simulink subsystem "NoVCU"  (R2024a)
settings: Solver=VariableStepAuto  StartTime=0.0  StopTime=10.0  RelTol=1e-3
settings Model: Creator=The MathWorks, Inc.  LastModifiedBy=The MathWorks, Inc.
settings RTWCC: GPUComputeCapability=3.5

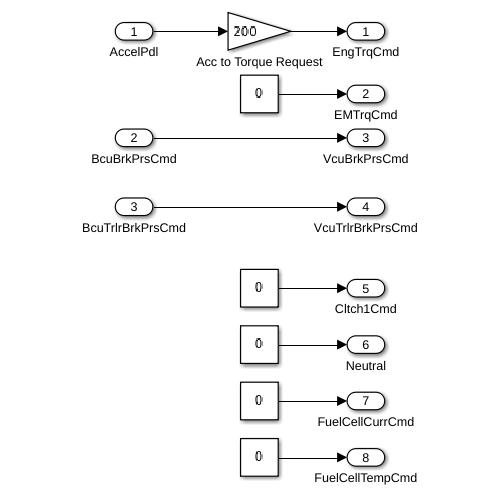
[thumbnail: Simulink's stored preview of the top-level diagram]
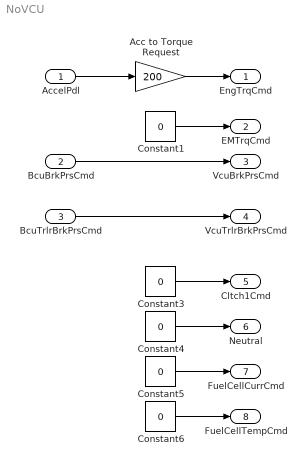
== system NoVCU ==
  AccelPdl : Inport
  BcuBrkPrsCmd : Inport  Port=2  SampleTime=0.01
  BcuTrlrBrkPrsCmd : Inport  Port=3  SampleTime=0.01
  Acc to Torque Request : Gain  Gain=200
  Constant{1,3..6} (5 alike) : Constant  Value=0  SampleTime=0.01
  EngTrqCmd : Outport  OutDataTypeStr=double  PortDimensions=1  SampleTime=[0.01,0]  VectorParamsAs1DForOutWhenUnconnected=off
  EMTrqCmd : Outport  Port=2  VectorParamsAs1DForOutWhenUnconnected=off
  VcuBrkPrsCmd : Outport  Port=3  PortDimensions=4  VectorParamsAs1DForOutWhenUnconnected=off
  VcuTrlrBrkPrsCmd : Outport  Port=4  PortDimensions=6  VectorParamsAs1DForOutWhenUnconnected=off
  Cltch1Cmd : Outport  Port=5  PortDimensions=1  SampleTime=[0.01,0]  VectorParamsAs1DForOutWhenUnconnected=off
  Neutral : Outport  Port=6  PortDimensions=1  SampleTime=[0.01,0]  VectorParamsAs1DForOutWhenUnconnected=off
  FuelCellCurrCmd : Outport  Port=7  SampleTime=.01
  FuelCellTempCmd : Outport  Port=8
  wires:
  Acc to Torque Request/1 -> EngTrqCmd/1
  Constant1/1 -> EMTrqCmd/1
  Constant3/1 -> Cltch1Cmd/1
  Constant4/1 -> Neutral/1
  Constant5/1 -> FuelCellCurrCmd/1
  Constant6/1 -> FuelCellTempCmd/1
  AccelPdl/1 -> Acc to Torque Request/1
  BcuBrkPrsCmd/1 -> VcuBrkPrsCmd/1
  BcuTrlrBrkPrsCmd/1 -> VcuTrlrBrkPrsCmd/1
